simulink subsystem "F550_PseudoInv_ControlAllocation"  (R2024a)
settings: Solver=VariableStepAuto  StartTime=0.0  StopTime=10.0  RelTol=1e-3
values from neighbouring files (symbols this model uses):
  Jxx = 0.00915    [F550_data.m]
  Jyy = 0.00915    [F550_data.m]
  Jzz = 0.01187    [F550_data.m]
  Mass = 2.06    [F550_data.m]
settings Model: Creator=UASG  LastModifiedBy=UASG

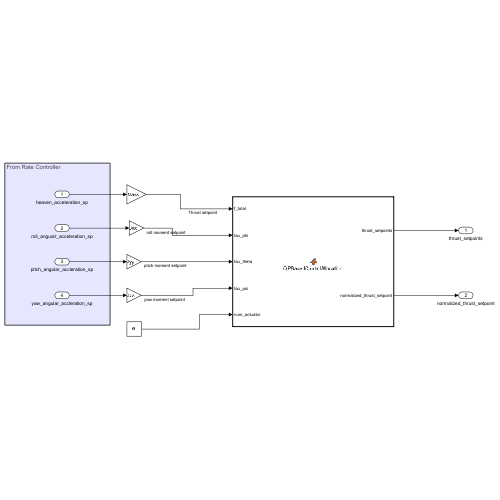
[thumbnail: Simulink's stored preview of the top-level diagram]
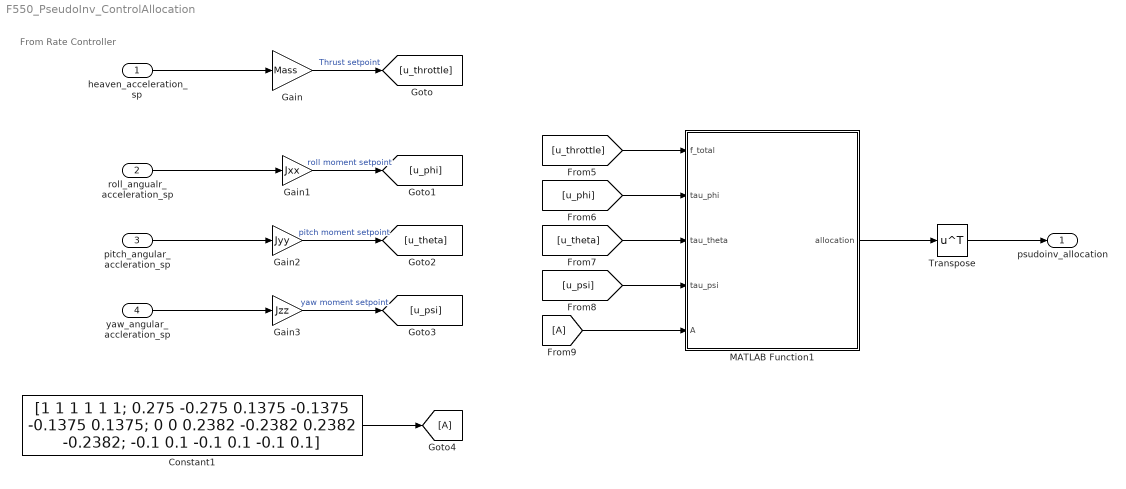
== system F550_PseudoInv_ControlAllocation ==
  note: From Rate Controller
  heaven_acceleration_sp : Inport
  roll_angualr_acceleration_sp : Inport  Port=2
  pitch_angular_accleration_sp : Inport  Port=3
  yaw_angular_accleration_sp : Inport  Port=4
  Constant1 : Constant  Value=[1 1 1 1 1 1; 0.275 -0.275 0.1375 -0.1375 -0.1375 0.1375; 0 0 0.2382 -0.2382 0.2382 -0.2382; -0.1 0.1 -0.1 0.1 -0.1 0.1]
  From9 : From
  Gain : Gain  Gain=Mass
  Gain1 : Gain  Gain=Jxx
  Gain2 : Gain  Gain=Jyy
  Gain3 : Gain  Gain=Jzz
  Goto4 : Goto
  MATLAB Function1 : MATLAB Function  TreatAsAtomicUnit=on
  Transpose : Math  Operator=transpose
  psudoinv_allocation : Outport
  wires:
  heaven_acceleration_sp/1 -> Gain/1
  roll_angualr_acceleration_sp/1 -> Gain1/1
  pitch_angular_accleration_sp/1 -> Gain2/1
  yaw_angular_accleration_sp/1 -> Gain3/1
  Constant1/1 -> Goto4/1
  Transpose/1 -> psudoinv_allocation/1
  Gain/1 -> [u_throttle]  "Thrust setpoint"
  Gain1/1 -> [u_phi]  "roll moment setpoint"
  Gain2/1 -> [u_theta]  "pitch moment setpoint"
  Gain3/1 -> [u_psi]  "yaw moment setpoint"
  From9/1 -> MATLAB Function1/5(A)
  [u_throttle] -> MATLAB Function1/1(f_total)
  [u_phi] -> MATLAB Function1/2(tau_phi)
  [u_theta] -> MATLAB Function1/3(tau_theta)
  [u_psi] -> MATLAB Function1/4(tau_psi)
  MATLAB Function1/1(allocation) -> Transpose/1

== matlab function F550_PseudoInv_ControlAllocation/MATLAB Function1 ==
  data: f_total input; allocation output; tau_phi input; tau_theta input; tau_psi input; A input
function allocation = PsuedoInvControlAllocation(f_total, tau_phi, tau_theta, tau_psi, A)


u_des = [f_total; tau_phi; tau_theta; tau_psi];
psudoinv = pinv(A);
allocation = psudoinv * u_des;
